simulink model "simulation_v1"  (R2025a)
settings: Solver=VariableStepAuto  StartTime=0.0  StopTime=10.0  RelTol=1e-3
undefined symbols (not defined in the file or in its folder): params
settings Model: Creator=dperera  LastModifiedBy=dperera

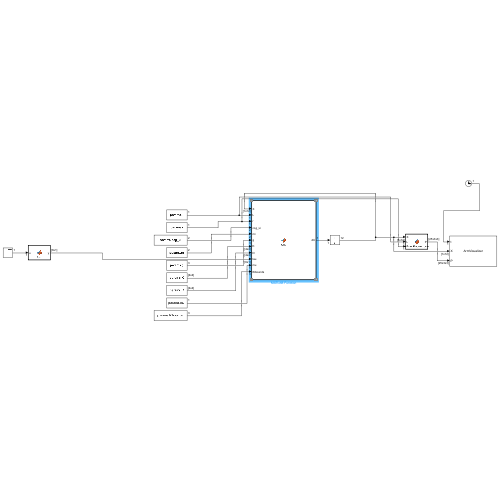
[thumbnail: Simulink's stored preview of the top-level diagram]
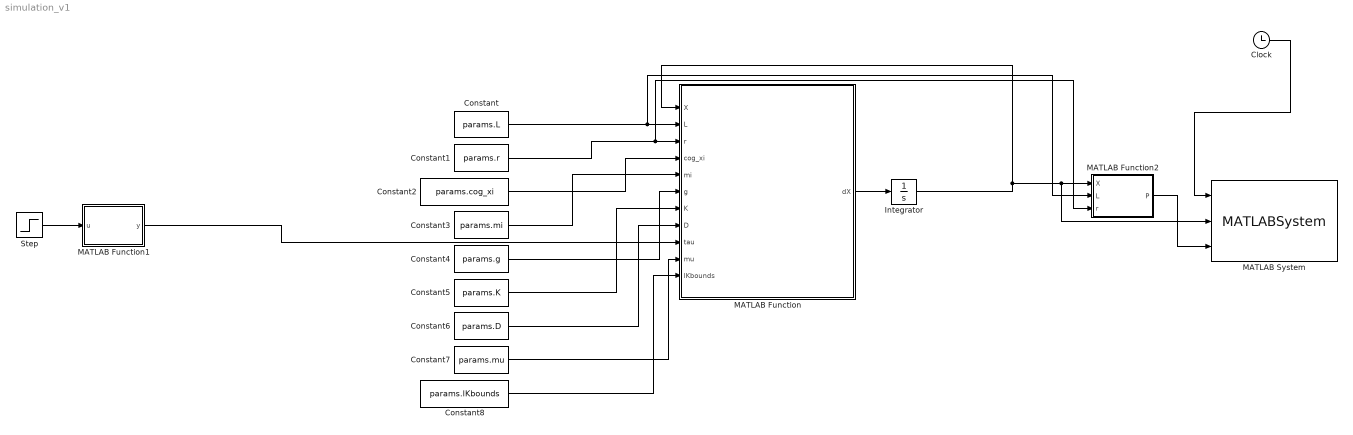
== system simulation_v1 ==
  Clock : Clock
  Constant : Constant  Value=params.L
  Constant1 : Constant  Value=params.r
  Constant2 : Constant  Value=params.cog_xi
  Constant3 : Constant  Value=params.mi
  Constant4 : Constant  Value=params.g
  Constant5 : Constant  Value=params.K
  Constant6 : Constant  Value=params.D
  Constant7 : Constant  Value=params.mu
  Constant8 : Constant  Value=params.lKbounds
  Integrator : Integrator  InitialCondition=[0;0;0;0;0;0;0;0;0;0;0;0]
  MATLAB Function : MATLAB Function  TreatAsAtomicUnit=on
  MATLAB Function1 : MATLAB Function  TreatAsAtomicUnit=on
  MATLAB Function2 : MATLAB Function  TreatAsAtomicUnit=on
  MATLAB System : MATLABSystem  System=ArmVisualizer  N=3  Nx=25  UseFlipZ=true  ShowStateLines=true  SimulateUsing=Code generation
      mask Type: ArmVisualizer
  Step : Step  SampleTime=0
  wires:
  Constant/1 -> MATLAB Function2/2(L), MATLAB Function/2(L)
  Constant1/1 -> MATLAB Function2/3(r), MATLAB Function/3(r)
  Constant2/1 -> MATLAB Function/4(cog_xi)
  Constant3/1 -> MATLAB Function/5(mi)
  Constant4/1 -> MATLAB Function/6(g)
  Constant5/1 -> MATLAB Function/7(K)
  Constant6/1 -> MATLAB Function/8(D)
  Constant7/1 -> MATLAB Function/10(mu)
  MATLAB Function/1(dX) -> Integrator/1
  Constant8/1 -> MATLAB Function/11(lKbounds)
  Step/1 -> MATLAB Function1/1(u)
  MATLAB Function1/1(y) -> MATLAB Function/9(tau)
  MATLAB Function2/1(P) -> MATLAB System/3
  Clock/1 -> MATLAB System/1
  Integrator/1 -> MATLAB System/2, MATLAB Function2/1(X), MATLAB Function/1(X)

== matlab function simulation_v1/MATLAB Function1 ==
  data: u input; y output
function y = fcn(u)
A = pi*(0.013/2)^2;
y = -(A * u * 1e5)*ones(6,1);

== matlab function simulation_v1/MATLAB Function ==
  data: dX output; X input; L input; r input; cog_xi input; mi input; g input; K input; D input; tau input; mu input; lKbounds input
function dX = fcn(X, L, r, cog_xi, mi, g, K, D, tau, mu, lKbounds)
%#codegen
t = 0;
dX = armS_dynamics_N3_entry_mex_mex(t, X, L, r, cog_xi, mi, g, K, D, tau, mu, lKbounds);
end

== matlab function simulation_v1/MATLAB Function2 ==
  data: X input; P output; L input; r input
function P = arm_backbone_points(X, L, r)
%#codegen
% Output P: [Nx x 3 x N], global points for each section backbone

N  = 3;
Nx = 25;

% fixed xi grid
xi = coder.const(linspace(0,1,Nx));

useFlipZ = true;

% unpack l (N x 2)
l_mat = reshape(X(1:2*N), [2, N]).'; % [N x 2]

Rglob = eye(3);
Pglob = zeros(3,1);

P = zeros(Nx,3,N);

for s = 1:N
    length_s = [0, l_mat(s,1), l_mat(s,2)];

    for j = 1:Nx
        % HTM_nume_mex must be codegen-compatible (it is a MEX; if not, replace with codegen version)
        [~, ~, Ploc] = HTM_nume_mex(length_s, xi(j), L, r);

        Ppoint = Pglob + Rglob * Ploc;

        if useFlipZ
            Ppoint = [1 0 0; 0 -1 0; 0 0 -1] * Ppoint;
        end

        P(j,1,s) = Ppoint(1);
        P(j,2,s) = Ppoint(2);
        P(j,3,s) = Ppoint(3);
    end

    % advance transforms (UNFLIPPED)
    [~, Rtip, Ptip] = HTM_nume_mex(length_s, 1, L, r);
    Pglob = Pglob + Rglob * Ptip;
    Rglob = Rglob * Rtip;
end
end
